simulink model "mass_sim_controller"  (R2015a)
settings: Solver=ode45  StartTime=0.0  StopTime=200  RelTol=1e-3
InitFcn:
  | param
undefined symbols (not defined in the file or in its folder): AP, drawMassSpringDamper, mass_ctrl, P
settings Model: Creator=beard  LastModifiedBy=ecestudent
settings DataIOCC: SignalLoggingSaveFormat=ModelDataLogs
settings OptimizationCC: ExpressionDepthLimit=2147483647  InitFltsAndDblsToZero=on
settings DebuggingCC: UnderspecifiedInitializationDetection=Classic  MergeDetectMultiDrivingBlocksExec=none  SolverPrmCheckMsg=warning  FcnCallInpInsideContextMsg=UseLocalSettings  StateNameClashWarn=warning
settings SFSimCC: SimCustomInitializer=param
settings GRTTargetCC: CombineOutputUpdateFcns=off  GRTInterface=on

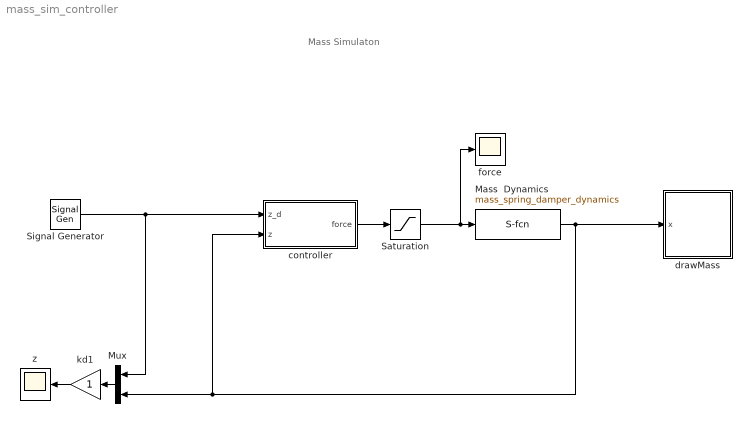
== system mass_sim_controller ==
  note: Mass Simulaton
  Mass  Dynamics : S-Function  FunctionName=mass_spring_damper_dynamics  Parameters=AP
  Mux : Mux  Inputs=2
  Saturation : Saturate  UpperLimit=P.F_max  LowerLimit=-P.F_max
  Signal Generator : SignalGenerator  WaveForm=square  Frequency=.02
  controller : Subsystem
  drawMass : Subsystem
      mask Display: image(imread('tv.jpg'))
  force : Scope
      settings: YMin=0.15  YMax=1
  kd1 : Gain
  z : Scope
      settings: TimeRange=40  YMin=-1  YMax=0.7
  wires:
  Signal Generator/1 -> Mux/1, controller/1(z_d)
  Mass  Dynamics/1 -> controller/2(z), Mux/2, drawMass/1(x)
  Mux/1 -> kd1/1
  kd1/1 -> z/1
  Saturation/1 -> Mass  Dynamics/1, force/1
  controller/1(force) -> Saturation/1

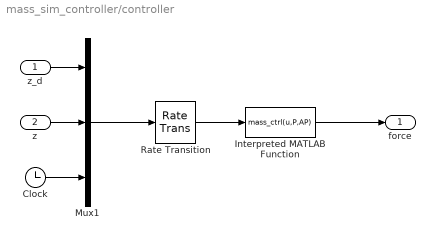
== system mass_sim_controller/controller ==
  z_d : Inport
  z : Inport  Port=2
  Clock : Clock
  Interpreted MATLAB Function : MATLABFcn  MATLABFcn=mass_ctrl(u,P,AP)  OutputDimensions=1
  Mux1 : Mux  Inputs=3
  Rate Transition : RateTransition  OutPortSampleTime=P.Ts
  force : Outport
  wires:
  Mux1/1 -> Rate Transition/1
  z_d/1 -> Mux1/1
  z/1 -> Mux1/2
  Interpreted MATLAB Function/1 -> force/1
  Clock/1 -> Mux1/3
  Rate Transition/1 -> Interpreted MATLAB Function/1

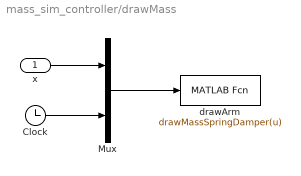
== system mass_sim_controller/drawMass ==
  x : Inport
  Clock : Clock
  Mux : Mux  Inputs=2
  drawArm : MATLABFcn  MATLABFcn=drawMassSpringDamper(u)  OutputDimensions=0  SampleTime=0.1
  wires:
  Mux/1 -> drawArm/1
  x/1 -> Mux/1
  Clock/1 -> Mux/2
